simulink model "Exemplu_figura5"  (R2016a)
settings: Solver=VariableStepDiscrete  StartTime=0.0  StopTime=20  RelTol=1e-3
settings Model: Creator=Cristina  LastModifiedBy=Cristina

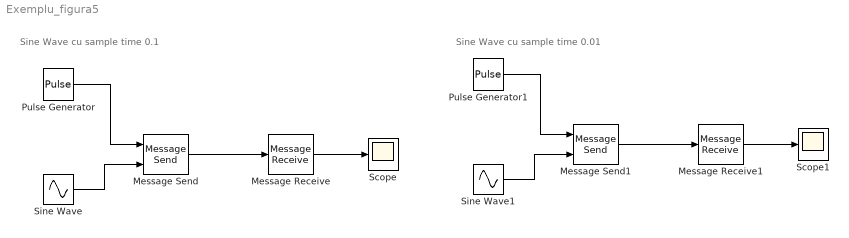
== system Exemplu_figura5 ==
  note: Sine Wave cu sample time 0.01
  note: Sine Wave cu sample time 0.1
  Message Receive : MessageReceive  InputPortMessageModes=m
      settings: OutputPortMap=o1
  Message Receive1 : MessageReceive  InputPortMessageModes=m
      settings: OutputPortMap=o1
  Message Send : MessageSend  OutputPortMessageModes=m  ShowEnablePort=on
      settings: InputPortMap=e0,u1
  Message Send1 : MessageSend  OutputPortMessageModes=m  ShowEnablePort=on
      settings: InputPortMap=e0,u1
  Pulse Generator : DiscretePulseGenerator  PulseType=Time based  Period=2*pi  PulseWidth=50
  Pulse Generator1 : DiscretePulseGenerator  PulseType=Time based  Period=2*pi  PulseWidth=50
  Scope : Scope
  Scope1 : Scope
  Sine Wave : Sin  Frequency=2  SampleTime=0.1
  Sine Wave1 : Sin  Frequency=2  SampleTime=0.01
  wires:
  Pulse Generator/1 -> Message Send/1
  Sine Wave/1 -> Message Send/2
  Message Send/1 -> Message Receive/1
  Message Receive/1 -> Scope/1
  Pulse Generator1/1 -> Message Send1/1
  Sine Wave1/1 -> Message Send1/2
  Message Send1/1 -> Message Receive1/1
  Message Receive1/1 -> Scope1/1
